simulink model "MIMO_linearized_simulink_model"  (R2017b)
settings: Solver=VariableStepAuto  StartTime=0.0  StopTime=270  RelTol=1e-3
values from neighbouring files (symbols this model uses):
  A = [dh1dh1 dh1dh2; dh2dh1 dh2dh2]    [SSV_milan.m]    (also in identifikace.m = -0.066; linear_systim.m)
  B = [ dh1du dh1dvt dh1dvo; dh2du dh2dvt dh2dvo ]    [SSV_milan.m]    (also in identifikace.m = -0.0144; linear_systim.m)
  C = [1 0; 0 1]    [SSV_milan.m]    (also in identifikace.m = -0.02; linear_systim.m)
  D = [ 0 0 0; 0 0 0]    [SSV_milan.m]    (also in linear_systim.m)
settings Model: Creator=ladislav  LastModifiedBy=ladislav

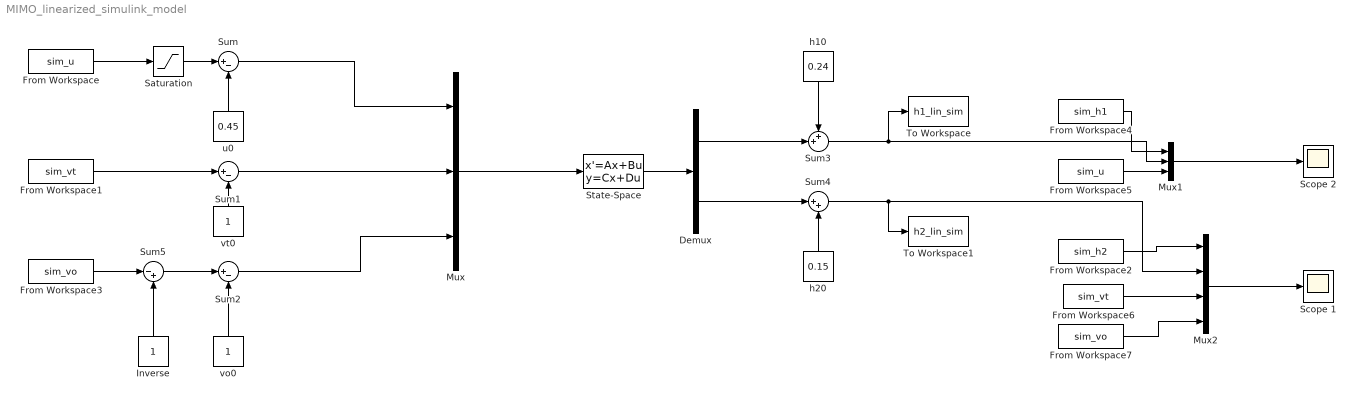
== system MIMO_linearized_simulink_model ==
  " Inverse " : Constant
  Demux : Demux  Outputs=2
  From Workspace : FromWorkspace  VariableName=sim_u  SampleTime=0
  From Workspace1 : FromWorkspace  VariableName=sim_vt  SampleTime=0
  From Workspace2 : FromWorkspace  VariableName=sim_h2  SampleTime=0
  From Workspace3 : FromWorkspace  VariableName=sim_vo  SampleTime=0
  From Workspace4 : FromWorkspace  VariableName=sim_h1  SampleTime=0
  From Workspace5 : FromWorkspace  VariableName=sim_u  SampleTime=0
  From Workspace6 : FromWorkspace  VariableName=sim_vt  SampleTime=0
  From Workspace7 : FromWorkspace  VariableName=sim_vo  SampleTime=0
  Mux : Mux  Inputs=3
  Mux1 : Mux  Inputs=3
  Mux2 : Mux
  "Saturation " : Saturate  UpperLimit=1
  Scope 1 : Scope
  Scope 2 : Scope
  State-Space : StateSpace  A=A  B=B  C=C  D=D  InitialCondition=0
  Sum : Sum  Inputs=|+-
  Sum1 : Sum  Inputs=|+-
  Sum2 : Sum  Inputs=|+-
  Sum3 : Sum  Inputs=++|
  Sum4 : Sum  Inputs=|++
  Sum5 : Sum  Inputs=|-+
  To Workspace : ToWorkspace  VariableName=h1_lin_sim  SaveFormat=Timeseries  SampleTime=-1
  To Workspace1 : ToWorkspace  VariableName=h2_lin_sim  SaveFormat=Timeseries  SampleTime=-1
  h10 : Constant  Value=0.24
  h20 : Constant  Value=0.15
  u0 : Constant  Value=0.45
  vo0 : Constant
  vt0 : Constant
  wires:
  u0/1 -> Sum/2
  From Workspace/1 -> "Saturation "/1
  vt0/1 -> Sum1/2
  From Workspace1/1 -> Sum1/1
  vo0/1 -> Sum2/2
  Sum1/1 -> Mux/2
  Sum/1 -> Mux/1
  Sum2/1 -> Mux/3
  Mux/1 -> State-Space/1
  h20/1 -> Sum4/2
  State-Space/1 -> Demux/1
  h10/1 -> Sum3/1
  Sum3/1 -> To Workspace/1, Mux1/2
  Sum4/1 -> Mux2/2, To Workspace1/1
  From Workspace3/1 -> Sum5/1
  " Inverse "/1 -> Sum5/2
  Sum5/1 -> Sum2/1
  Mux1/1 -> Scope 2/1
  From Workspace4/1 -> Mux1/1
  From Workspace5/1 -> Mux1/3
  Mux2/1 -> Scope 1/1
  From Workspace6/1 -> Mux2/3
  From Workspace2/1 -> Mux2/1
  Demux/2 -> Sum4/1
  Demux/1 -> Sum3/2
  "Saturation "/1 -> Sum/1
  From Workspace7/1 -> Mux2/4
